simulink model "Hw6P1b"  (R2017a)
settings: Solver=FixedStepAuto  StartTime=0.0  StopTime=10.0  FixedStep=0.01  RelTol=1e-3
settings Model: Creator=Soutrik  LastModifiedBy=Soutrik

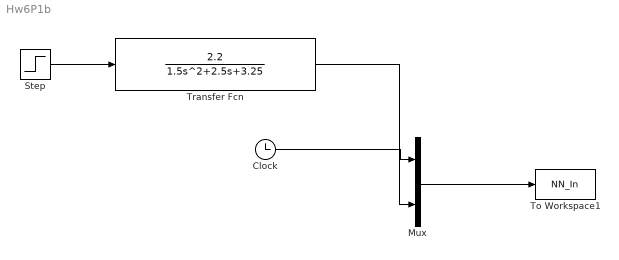
== system Hw6P1b ==
  Clock : Clock
  Mux : Mux  Inputs=2
  Step : Step  SampleTime=0
  To Workspace1 : ToWorkspace  VariableName=NN_In  SampleTime=-1
  Transfer Fcn : TransferFcn  Numerator=[2.2]  Denominator=[1.5 2.5 3.25]
  wires:
  Step/1 -> Transfer Fcn/1
  Clock/1 -> Mux/1
  Mux/1 -> To Workspace1/1
  Transfer Fcn/1 -> Mux/2
